simulink model "circuit7lk"  (Simulink 5.0)
settings: Solver=ode23tb  StartTime=0.0  StopTime=1.5  RelTol=1e-3
libraries: powerlib2 x7, powerlib_extras x2
settings Model: LastModifiedBy=User

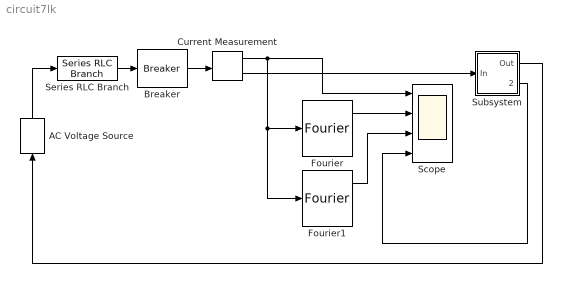
== system circuit7lk ==
  AC Voltage Source : powerlib2/Electrical Sources/AC Voltage Source  Tag=PoWeRsYsTeMbLoCk  Description=source block  Orientation=up  A=120*sqrt(2)  P=0  F=60  stime=0  mesure=None  PSBOutputType=1
  Breaker : powerlib2/Elements/Breaker  Tag=PoWeRsYsTeMbLoCk  a=0.01  c=0  rs=1e6  cs=inf  times=[ 1/60 ]  Ts=0  comext=off  mesure=None  PSBOutputType=1
  Current Measurement : powerlib2/Measurements/Current Measurement  Tag=PoWeRsYsTeMmEaSuReMeNt  PhasorSimulation=off  OutputType=Magnitude  PSBOutputType=01  PSBequivalent=0
  Fourier : powerlib_extras/Measurements/Fourier  f1=60  n=1
  Fourier1 : powerlib_extras/Measurements/Fourier  f1=60  n=0
  Scope : Scope  NumInputPorts=4
      settings: YMin=-5~-5~-5~-5  YMax=5~5~5~5
  Series RLC Branch : powerlib2/Elements/Series RLC Branch  Tag=PoWeRsYsTeMbLoCk  a=5  b=0  c=inf  mesure=None  PSBOutputType=1
  Subsystem : Subsystem  mask(Nonlinear Inductance){Vnom=120, fnom=60, L=2, sat=[0 0; 1 1; 2 1.25]}
      mask prompts: Vnom "Nominal voltage (Volts rms) :"; fnom "Nominal frequency (Hz):"; L "Unsaturated inductance (H):"; sat "Saturation characteristic [i1(pu) phi1(pu); i2 phi2; ...]:"
      mask init:
      | % Define base current and Flux for p.u. system
      | I_base=Vnom*sqrt(2)/(L*2*pi*fnom);
      | Phi_base=Vnom*sqrt(2)/(2*pi*fnom);
      | % Check first two points of the saturation characteristic
      | if ~all(all(sat(1:2,:)==[0 0; 1 1])),
      | h=errordlg('The first two points of the characteristic must be [0 0; 1 1]','Error');
      | uiwait(h);
      | end
      | % Complete negative part of saturation characteristic
      | [npoints,ncol]=size(sat);
      | sat1=[sat ; -sat(2:npoints,:)];
      | sat1=sort(sat1);
      | % Current vector (A) and flux vector (V.s)
      | Current_vect=sat1(:,1)*I_base;
      | Flux_vect=sat1(:,2)*Phi_base;
      mask Display: plot(Current_vect,Flux_vect)
  wires:
  AC Voltage Source/1 -> Series RLC Branch/1
  Series RLC Branch/1 -> Breaker/1
  Current Measurement/1 -> Fourier/1, Fourier1/1, Scope/1
  Current Measurement/2 -> Subsystem/1(In)
  Fourier/1 -> Scope/2
  Fourier1/1 -> Scope/3
  Subsystem/2(Flux) -> Scope/4
  Subsystem/1(Out) -> AC Voltage Source/1
  Breaker/1 -> Current Measurement/1

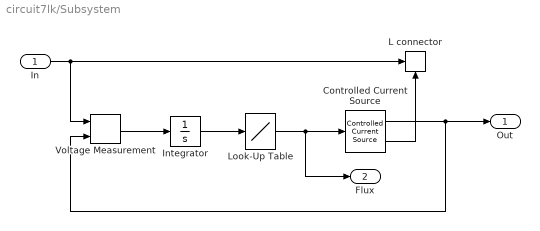
== system circuit7lk/Subsystem ==
  In : Inport
  Controlled Current Source : powerlib2/Electrical Sources/Controlled Current Source  Tag=PoWeRsYsTeMbLoCk  Description=source block  initsrc=on  srctyp=AC  ia=0  iph=0  freq=0  mesure=None  PSBOutputType=11
  Integrator : Integrator
  L connector : powerlib2/Connectors/L connector  Tag=PoWeRsYsTeMbLoCk  Orientation=up
  Look-Up Table : Lookup  InputValues=Flux_vect  OutputValues=Current_vect  SaturateOnIntegerOverflow=on
  Voltage Measurement : powerlib2/Measurements/Voltage Measurement  Tag=PoWeRsYsTeMmEaSuReMeNt  PhasorSimulation=off  OutputType=Magnitude  PSBOutputType=0  PSBequivalent=1
  Out : Outport
  Flux : Outport  Port=2
  wires:
  Voltage Measurement/1 -> Integrator/1
  Integrator/1 -> Look-Up Table/1
  Look-Up Table/1 -> Flux/1, Controlled Current Source/1
  In/1 -> L connector/Enable, Voltage Measurement/1
  Controlled Current Source/2 -> L connector/1
  Controlled Current Source/1 -> Voltage Measurement/2, Out/1
